simulink model "week2_force_model"  (R2025b)
settings: Solver=VariableStepAuto  StartTime=0.0  StopTime=10.0  RelTol=1e-3
settings Model: Creator=legob  LastModifiedBy=legob

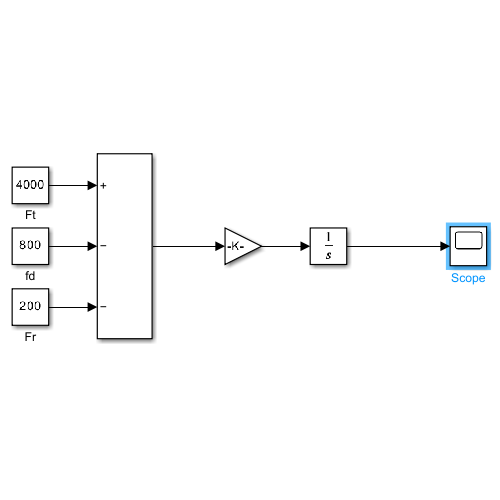
[thumbnail: Simulink's stored preview of the top-level diagram]
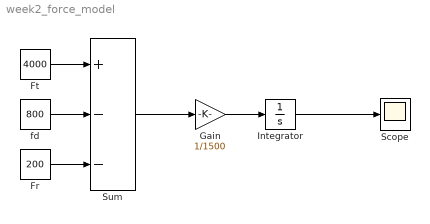
== system week2_force_model ==
  Fr : Constant  Value=200
  Ft : Constant  Value=4000
  Gain : Gain  Gain=1/1500
  Integrator : Integrator  InitialCondition=20
  Scope : Scope
      settings: ActiveDisplayYMinimum=17.500000000000007  ActiveDisplayYMaximum=42.499999999999929
  Sum : Sum  Inputs=+--
  fd : Constant  Value=800
  wires:
  Integrator/1 -> Scope/1
  Ft/1 -> Sum/1
  fd/1 -> Sum/2
  Fr/1 -> Sum/3
  Sum/1 -> Gain/1
  Gain/1 -> Integrator/1
